simulink model "ps4"  (R2015a)
settings: Solver=ode45  StartTime=0.0  StopTime=10.0  RelTol=1e-3
undefined symbols (not defined in the file or in its folder): A4, B4, C4, K_poleplace_1
settings Model: Creator=Sam  LastModifiedBy=Sam

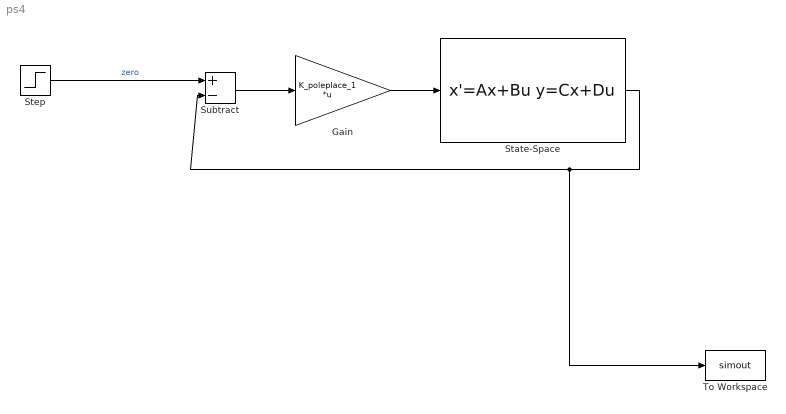
== system ps4 ==
  Gain : Gain  Gain=K_poleplace_1  Multiplication=Matrix(K*u)
  State-Space : StateSpace  A=A4  B=B4  C=C4  D=B4*0  X0=[ 0, 0, 1.5, 0, 0, 0, 0, 0, 0, 0, 0, 0]
  Step : Step  Before=[ 0, 0, 0, 0, 0, 0, 0, 0, 0, 0, 0, 0]  After=[ 0, 0, 0, 0, 0, 0, 0, 0, 0, 0, 0, 0]  SampleTime=0
  Subtract : Sum  Inputs=+-
  To Workspace : ToWorkspace  VariableName=simout  SaveFormat=Timeseries  SampleTime=-1
  wires:
  State-Space/1 -> To Workspace/1, Subtract/2
  Subtract/1 -> Gain/1
  Gain/1 -> State-Space/1
  Step/1 -> Subtract/1  "zero"
